simulink model "sensors_subsystem"  (R2024a)
settings: Solver=VariableStepAuto  StartTime=0.0  StopTime=10.0  RelTol=1e-3
undefined symbols (not defined in the file): Acel_X, Acel_Y, Acel_Z, Cam_Left_Orientation, Cam_Left_Position, Cam_Right_Orientation, Cam_Right_Position, Gyro_X, Gyro_Y, Gyro_Z, Hydrophone_Bearing, Hydrophone_Distance, Leak_Detected, Pressure_Pa
libraries: simulink x9
settings Model: Creator=adity  LastModifiedBy=adity

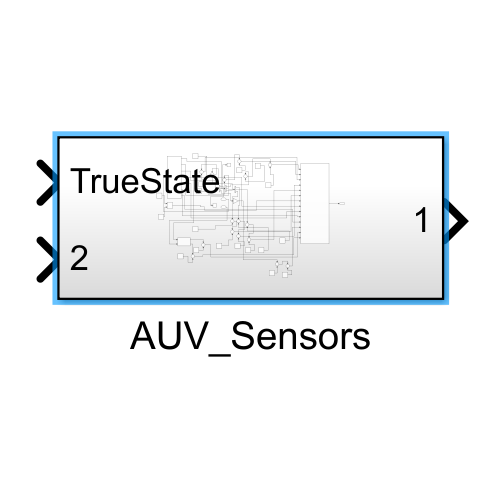
[thumbnail: Simulink's stored preview of the top-level diagram]
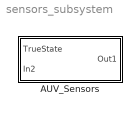
== system sensors_subsystem ==
  AUV_Sensors : Subsystem

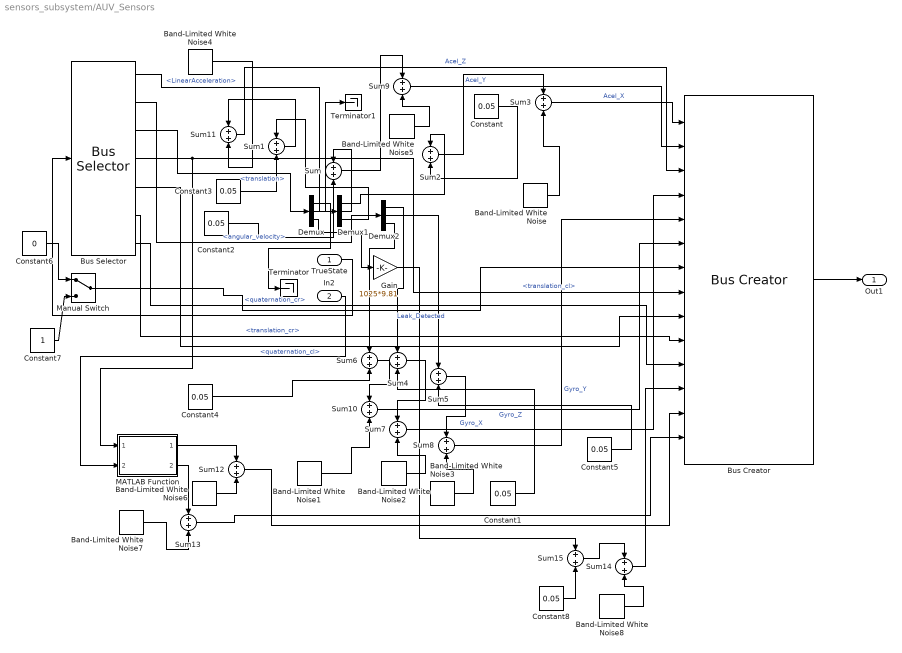
== system sensors_subsystem/AUV_Sensors ==
  TrueState : Inport
  In2 : Inport  Port=2
  Band-Limited White Noise{,1..8} (9 alike) : simulink/Sources/Band-Limited White Noise  Cov=[0.1]  Ts=0.1  seed=[23341]
  Bus Creator : BusCreator  Inputs=Acel_X,Acel_Y,Acel_Z,Gyro_X,Gyro_Y,Gyro_Z,Leak_Detected,Cam_Left_Position,Cam_Left_Orientation,Cam_Right_Position,Cam_Right_Orientation,Pressure_Pa,Hydrophone_Distance,Hydrophone_Bearing
  Bus Selector : BusSelector  OutputSignals=LinearAcceleration,angular_velocity,translation,translation_cl,quaternation_cl,translation_cr,quaternation_cr
  Constant{,1..5,8} (7 alike) : Constant  Value=0.05
  Constant6 : Constant  Value=0
  Constant7 : Constant
  Demux : Demux  Outputs=3
  Demux1 : Demux  Outputs=3
  Demux2 : Demux  Outputs=3
  Gain : Gain  Gain=1025*9.81
  MATLAB Function : MATLAB Function  TreatAsAtomicUnit=on
  Manual Switch : ManualSwitch
  Sum{,1..15} (16 alike) : Sum
  Terminator : Terminator
  Terminator1 : Terminator
  Out1 : Outport
  wires:
  TrueState/1 -> Bus Selector/1
  Bus Creator/1 -> Out1/1
  Bus Selector/3 -> Demux/1  "<translation>"
  Bus Selector/1 -> Demux1/1  "<LinearAcceleration>"
  Bus Selector/2 -> Demux2/1  "<angular_velocity>"
  Demux/3 -> Gain/1
  Demux1/1 -> Sum2/1
  Constant/1 -> Sum2/2
  Sum2/1 -> Sum3/1
  Band-Limited White Noise/1 -> Sum3/2
  Demux1/2 -> Sum/1
  Demux1/3 -> Sum1/1
  Demux2/1 -> Sum4/1
  Demux2/2 -> Sum5/1
  Demux2/3 -> Sum6/1
  Constant4/1 -> Sum6/2
  Constant3/1 -> Sum1/2
  Constant2/1 -> Sum/2
  Constant1/1 -> Sum4/2
  Constant5/1 -> Sum5/2
  Sum1/1 -> Sum11/1
  Sum/1 -> Sum9/1
  Sum6/1 -> Sum10/1
  Sum4/1 -> Sum7/1
  Sum5/1 -> Sum8/1
  Band-Limited White Noise1/1 -> Sum10/2
  Band-Limited White Noise2/1 -> Sum7/2
  Band-Limited White Noise3/1 -> Sum8/2
  Band-Limited White Noise4/1 -> Sum11/2
  Band-Limited White Noise5/1 -> Sum9/2
  Sum3/1 -> Bus Creator/1  "Acel_X"
  Sum9/1 -> Bus Creator/2  "Acel_Y"
  Sum11/1 -> Bus Creator/3  "Acel_Z"
  Sum7/1 -> Bus Creator/4  "Gyro_X"
  Sum8/1 -> Bus Creator/5  "Gyro_Y"
  Sum10/1 -> Bus Creator/6  "Gyro_Z"
  Constant6/1 -> Manual Switch/1
  Constant7/1 -> Manual Switch/2
  Manual Switch/1 -> Bus Creator/7  "Leak_Detected"
  Bus Selector/4 -> Bus Creator/8, MATLAB Function/1(auv_pos)  "<translation_cl>"
  Bus Selector/5 -> Bus Creator/9  "<quaternation_cl>"
  Bus Selector/6 -> Bus Creator/10  "<translation_cr>"
  Bus Selector/7 -> Bus Creator/11  "<quaternation_cr>"
  In2/1 -> MATLAB Function/2(beacon_pos)
  MATLAB Function/1(distance) -> Sum12/1
  Band-Limited White Noise6/1 -> Sum12/2
  Band-Limited White Noise7/1 -> Sum13/2
  MATLAB Function/2(bearing) -> Sum13/1
  Sum12/1 -> Bus Creator/13
  Sum13/1 -> Bus Creator/14
  Gain/1 -> Sum15/1
  Constant8/1 -> Sum15/2
  Sum15/1 -> Sum14/1
  Band-Limited White Noise8/1 -> Sum14/2
  Sum14/1 -> Bus Creator/12
  Demux/1 -> Terminator/1
  Demux/2 -> Terminator1/1

== matlab function sensors_subsystem/AUV_Sensors/MATLAB Function ==
  data: auv_pos input; distance output; beacon_pos input; bearing output
function [distance, bearing] = fcn(auv_pos, beacon_pos)
% This function calculates the distance and bearing from the AUV to a beacon.

% Calculate the vector from the AUV to the beacon
vector_to_beacon = beacon_pos - auv_pos;

% Calculate the 3D distance (magnitude of the vector)
distance = sqrt(vector_to_beacon(1)^2 + vector_to_beacon(2)^2 + vector_to_beacon(3)^2);

% Calculate the bearing (the angle in the horizontal X-Y plane)
% atan2 is used to get the correct angle from -pi to +pi
bearing = atan2(vector_to_beacon(2), vector_to_beacon(1));

end
